simulink model "mars_rover_ex_3_22b"  (R2022b)
settings: Solver=ode23t  StartTime=0.0  StopTime=Rover.simStopTimeEx3  FixedStep=1e-2  MaxStep=0.05  RelTol=1e-3  AbsTol=1e-3  EnableMultiTasking=on
StartFcn:
  | setMechExplorerVisibility(bdroot,'hide');
  | mars_rover_ex3_sim_callback
StopFcn:
  | setMechExplorerVisibility(bdroot,'show');
model workspace (MATLAB code in the model file):
  | addpath("mars_rover_helpers");
  | % Load Rover Arm model for IK
  | mdlpath = ['mars_rover_data',filesep,'mars_rover_arm'];
  | load_system(mdlpath);
  | 
  | imdata = zeros(3,3,3);
  | 
  | % Temp
  | Kp_steer = 1;
  | Ki_steer = 1;
  | Kd_steer = 1;
  | 
  | Kp = 1;
  | Ki = 1;
  | Kd = 1;
values from neighbouring files (symbols this model uses):
  cam_base_angle = 0    [mars_rover_params.m]
  cam_target_angle = 20    [mars_rover_params.m]
  mapData = false(197,200)    [mars_rover_params.m]    (also in mars_rover_startup.m)
  roverPath = app.rover_path    [NavigateOnMars.m]    (also in mars_rover_params.m = rover_path1)
undefined symbols (not defined in the file or in its folder): Arm, armJointAng, armJointTrqs, cameraData, eeConfig, pose, Rover, sampleLocation, steerAng, steerTrqs, Terrain, vSpeed, Wheel1_G, Wheel2_G, Wheel3_G, Wheel4_G, Wheel5_G, Wheel6_G, wheelTrqs, wSpeeds, X, Y, Z
libraries: sm_lib x238, nesl_utility x80, slpidlib x3, simulink x3, simulink_extras x2, robotcorelib x1, robotalgslib x1
(part 1 of 9)
settings Model: PacingRate=4  Creator=The MathWorks, Inc.  LastModifiedBy=hupadhya
settings SolverCC: AutoScaleAbsTol=off  ZeroCrossAlgorithm=Adaptive  AlgebraicLoopSolver=TrustRegion  MinimalZcImpactIntegration=on  MaxZcPerStep=1
settings DataIOCC: MaxDataPoints=10000  SaveFormat=Array  ReturnWorkspaceOutputsName=sm_mars_rover_out_ex3
settings OptimizationCC: LifeSpan=inf
settings DebuggingCC: IgnoredZcDiagnostic=none  UnconnectedInputMsg=warning  UnconnectedOutputMsg=warning  UnconnectedLineMsg=warning  AllowSymbolicDim=off  SFUnexpectedBacktrackingDiag=warning  SFNoUnconditionalDefaultTransitionDiag=warning  SFExecutionAtInitializationDiag=none  SFMachineParentedDataDiag=warning  ArithmeticOperatorsInVariantConditions=warning
settings ModelReferenceCC: EnableRefExpFcnMdlSchedulingChecks=on
settings SFSimCC: SimUseLocalCustomCode=off  CustomCodeUndefinedFunction=UseInterfaceOnly
settings RTWCC: RTWUseLocalCustomCode=off  DLArmComputeVersion=19.05
settings CodeAppCC: StateflowObjectComments=on
settings GRTTargetCC: TargetLangStandard=C89/C90 (ANSI)
settings ConfigComp: CovMetricSettings=dw  CovSaveCumulativeToWorkspaceVar=on  CovSaveSingleToWorkspaceVar=on  CovExternalEMLEnable=off  CovSFcnEnable=off
settings SimscapeCC: SimscapeLogType=all  SimscapeLogSimulationStatistics=on  SimscapeLogName=simlog_sm_mars_rover  SimscapeLogLimitData=off  SimscapeLogDataHistory=10000
settings DiagnosticsConfigSet: SimMechanicsConflictingReferenceFrames=none
settings ExplorerConfigSet: InternalSimMechanicsExplorerSettings="<ExplorerConfiguration><canonicalview>default</canonicalview><AnimationSetting><BasePlaybackSpeed>1.0</BasePlaybackSpeed><PlaybackSpeedFactor>32.0</PlaybackSpeedFactor></AnimationSetting><TilePanel><TileInfo><Tiles Columns=\"1\" Count=\"1\" Rows=\"1\"><Column Weight=\"1\"/><Row Weight=\"1\"/><Tile Height=\"1\" Width=\"1\" X=\"0\" Y=\"0\"/></Tiles></TileInfo><SceneInfo><SceneViewer><BGColor><R>0.819607853889465332</R><G>0.709803938865661621</G><B>0.662745118141174316</B></BGColor><Camera><DoPerspective>off</DoPerspective><Position><X>20.000000787900472</X><Y>-8.56686066937523805</Y><Z>2.96310305518206007</Z></Position><Center><X>20.000000787900472</X><Y>19.6116538286981559</Y><Z>2.96310305518206007</Z></Center><Up><X>0</X><Y>-0</Y><Z>1</Z></Up><ViewLimDist>1</ViewLimDist><YLim>14.4034443168771542</YLim><XLim>20.6000000000000014</XLim></Camera></SceneViewer></SceneInfo></TilePanel><MechEditorPanel><Cameras><Camera><Id>Camera1</Id><Value><Name>Rover_Free_View</Name><NativeCamera><PositionKeyframeSet/><CenterKeyframeSet/><UpVectorKeyframeSet/></NativeCamera></Value></Camera><Camera><Id>Camera6</Id><Value><Name>Rover_Right_ViewA</Name><NativeCamera><PositionTrackingFeature>Mars_Rover.Rover_Plant_Model_And_Control.Rover.Chassis.Chasis_Camera_RightA.R</PositionTrackingFeature><CenterTrackingFeature>Mars_Rover.Rover_Plant_Model_And_Control.Rover.Chassis.Chasis_Camera_RightA.R</CenterTrackingFeature><UpVectorTrackingFeature>Mars_Rover.Rover_Plant_Model_And_Control.Rover.Chassis.Chasis_Camera_RightA.R</UpVectorTrackingFeature><CenterTrackingOrigin>off</CenterTrackingOrigin><CenterTrackingDirection>+X</CenterTrackingDirection><UpVectorTrackingDirection>+Z</UpVectorTrackingDirection></NativeCamera></Value></Camera><Camera><Id>Camera7</Id><Value><Name>Rover_Rear_View</Name><NativeCamera><PositionTrackingFeature>Mars_Rover.Rover_Plant_Model_And_Control.Rover.Chassis.Chasis_Camera_Rear.R</PositionTrackingFeature><CenterTrackingFeature>Mars_Rover.Rover_Plant_Model_And_Control.Rover.Chassis.Chasis_Camera_Rear.R</CenterTrackingFeature><UpVectorTrackingFeature>Mars_Rover.Rover_Plant_Model_And_Control.Rover.Chassis.Chasis_Camera_Rear.R</UpVectorTrackingFeature><CenterTrackingOrigin>off</CenterTrackingOrigin><CenterTrackingDirection>-Y</CenterTrackingDirection><UpVectorTrackingDirection>+Z</UpVectorTrackingDirection></NativeCamera></Value></Camera><Camera><Id>Camera8</Id><Value><Name>Rover_Top_View</Name><NativeCamera><PositionTrackingFeature>Mars_Rover.Rover_Plant_Model_And_Control.Rover.Chassis.Chasis_Camera_Top.R</PositionTrackingFeature><CenterTrackingFeature>Mars_Rover.Rover_Plant_Model_And_Control.Rover.Chassis.Chasis_Camera_Top.R</CenterTrackingFeature><UpVectorTrackingFeature>Mars_Rover.Rover_Plant_Model_And_Control.Rover.Chassis.Chasis_Camera_Top.R</UpVectorTrackingFeature><CenterTrackingOrigin>off</CenterTrackingOrigin><CenterTrackingDirection>-Z</CenterTrackingDirection><UpVectorTrackingDirection>+X</UpVectorTrackingDirection></NativeCamera></Value></Camera><Camera><Id>Camera9</Id><Value><Name>Rover_Right_ViewB</Name><NativeCamera><PositionTrackingFeature>Mars_Rover.Rover_Plant_Model_And_Control.Rover.Chassis.Chasis_Camera_RightB.R</PositionTrackingFeature><CenterTrackingFeature>Mars_Rover.Rover_Plant_Model_And_Control.Rover.Chassis.Chasis_Camera_RightB.R</CenterTrackingFeature><UpVectorTrackingFeature>Mars_Rover.Rover_Plant_Model_And_Control.Rover.Chassis.Chasis_Camera_RightB.R</UpVectorTrackingFeature><CenterTrackingOrigin>off</CenterTrackingOrigin><CenterTrackingDirection>+X</CenterTrackingDirection><UpVectorTrackingDirection>+Z</UpVectorTrackingDirection></NativeCamera></Value></Camera><Camera><Id>Camera10</Id><Value><Name>RoverNavCamL</Name><NativeCamera><PositionTrackingFeature>Mars_Rover.Rover_Plant_Model_And_Control.Rover.Camera.rsm_head_1_RIGID.CameraFrameL.F</PositionTrackingFeature><CenterTrackingFeature>Mars_Rover.Rover_Plant_Model_And_Control.Rover.Camera.rsm_head_1_RIGID.CameraFrameL.F</CenterTrackingFeature><UpVectorTrackingFeature>Mars_Rover.Rover_Plant_Model_And_Control.Rover.Camera.rsm_head_1_RIGID.CameraFrameL.F</UpVectorTrackingFeature><CenterTrackingOrigin>off</CenterTrackingOrigin><CenterTrackingDirection>+X</CenterTrackingDirection><UpVectorTrackingDirection>+Z</UpVectorTrackingDirection></NativeCamera></Value></Camera><Camera><Id>Camera11</Id><Value><Name>RoverNavCamR</Name><NativeCamera><PositionTrackingFeature>Mars_Rover.Rover_Plant_Model_And_Control.Rover.Camera.rsm_head_1_RIGID.CameraFrameR.F</PositionTrackingFeature><CenterTrackingFeature>Mars_Rover.Rover_Plant_Model_And_Control.Rover.Camera.rsm_head_1_RIGID.CameraFrameR.F</CenterTrackingFeature><UpVectorTrackingFeature>Mars_Rover.Rover_Plant_Model_And_Control.Rover.Camera.rsm_head_1_RIGID.CameraFrameR.F</UpVectorTrackingFeature><CenterTrackingOrigin>off</CenterTrackingOrigin><CenterTrackingDirection>+X</CenterTrackingDirection><UpVectorTrackingDirection>+Z</UpVectorTrackingDirection></NativeCamera></Value></Camera></Cameras><GfxPanelCameraMap/><VideoCreator><PlaybackSpeedRatio>8</PlaybackSpeedRatio><FrameRate>30</FrameRate><VideoFormat>MPEG-4</VideoFormat><FrameSize>[800 600]</FrameSize></VideoCreator></MechEditorPanel></ExplorerConfiguration>"

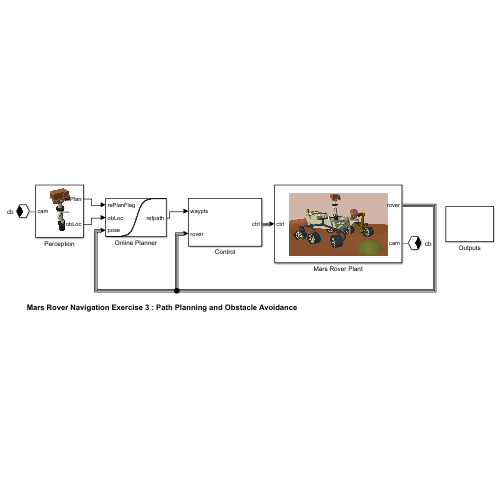
[thumbnail: Simulink's stored preview of the top-level diagram]
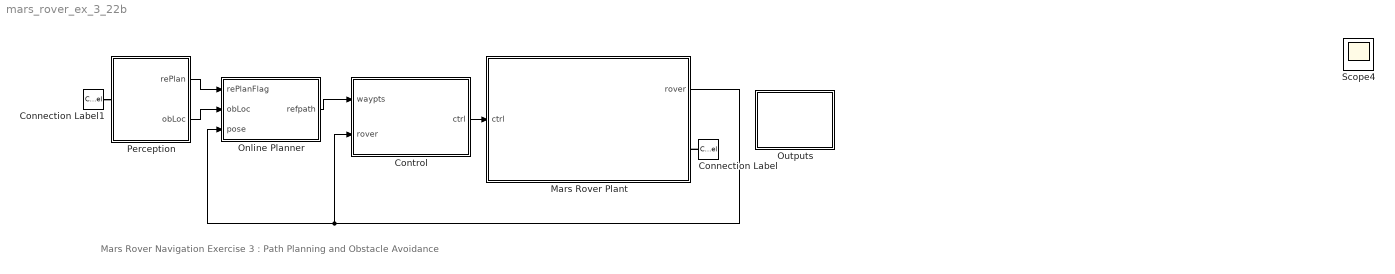
== system mars_rover_ex_3_22b ==
  note: Mars Rover Navigation Exercise 3 : Path Planning and Obstacle Avoidance
  Connection Label : ConnectionLabel  Label=cb
  Connection Label1 : ConnectionLabel  Label=cb
  Control : Subsystem
  Mars Rover Plant : Subsystem
      mask Display: image('$imagefile'); % Use "Edit Image" on toolstrip to change.
  Online Planner : Subsystem
      mask Display:
      | x = -5:0.01:5;
      | y = tanh(x);
      | plot(x,y)
  Outputs : Subsystem
  Perception : Subsystem
      mask Display: image('$imagefile'); % Use "Edit Image" on toolstrip to change.
  Scope4 : Scope
  wires:
  Mars Rover Plant/1(rover) -> Online Planner/3(pose), Control/2(rover)
  Control/1(ctrl) -> Mars Rover Plant/1(ctrl)
  Online Planner/1(refpath) -> Control/1(waypts)
  Perception/1(rePlan) -> Online Planner/1(rePlanFlag)
  Perception/2(obLoc) -> Online Planner/2(obLoc)
  connections:
  Connection Label/LConn1 -- Mars Rover Plant/RConn1
  Connection Label1/LConn1 -- Perception/LConn1

== system mars_rover_ex_3_22b/Control ==
  waypts : Inport
  rover : Inport  Port=2
  Bus Creator : BusCreator  Inputs=steerTrqs,wheelTrqs,armJointTrqs
  Bus Selector : BusSelector  OutputSignals=pose,vSpeed,steerAng,wSpeeds,sampleLocation,armJointAng
  Manipulator Control : Subsystem
  Rover Control : Subsystem
  ctrl : Outport
  wires:
  Bus Selector/3 -> Rover Control/4(ActSteerAng)  "<steerAng>"
  Bus Selector/6 -> Manipulator Control/2(ActJointAngles)  "<armJointAng>"
  Bus Selector/5 -> Manipulator Control/1(SampleLocation)  "<sampleLocation>"
  Bus Selector/2 -> Rover Control/3(vSpeed)  "<vSpeed>"
  Rover Control/2(WheelTrqs) -> Bus Creator/2  "wheelTrqs"
  Bus Selector/1 -> Rover Control/2(CurrentPose)  "<pose>"
  Bus Selector/4 -> Rover Control/5(ActWheelSpeed)  "<wSpeeds>"
  Rover Control/1(SteerTrqs) -> Bus Creator/1  "steerTrqs"
  Manipulator Control/1(y) -> Bus Creator/3  "armJointTrqs"
  rover/1 -> Bus Selector/1
  waypts/1 -> Rover Control/1(WayPts)
  Bus Creator/1 -> ctrl/1

== system mars_rover_ex_3_22b/Mars Rover Plant ==
  ctrl : Inport
  Bus Creator : BusCreator  Inputs=pose,vSpeed,steerAng,wSpeeds,armJointAng,sampleLocation
  Bus Selector : BusSelector  OutputSignals=steerTrqs,wheelTrqs,armJointTrqs
  DesRoverPathViz : Subsystem
  Manipulator Plant Model : Subsystem
      settings: PortSchema="{\"entries\":[{\"content\":{\"sides\":[{\"content\":{\"connectorIds\":[\"LConn1\",\"In1\"]},\"type\":\"ConnectorPlacement.EquallySpacedRectSide\",\"uuid\":\"1d5d5bba-8fe4-4512-81c9-941bf10e7a7e\"},{\"content\":{\"connectorIds\":[\"RConn1\",\"RConn2\",\"Out1\",\"Out2\"],\"side\":\"RIGHT\"},\"type\":\"ConnectorPlacement.EquallySpacedRectSide\",\"uuid\":\"9a182200-9de3-47d0-8b03-f46c5c0d90b9\"},{\"content\":{\"connectorIds\":[],\"side\":\"TOP\"},\"type\":\"ConnectorPlacement.EquallySpacedRectSide\",\"uuid\":\"d91c9a9a-8a5e-48c7-bbfb-96bbdec144af\"}]},\"type\":\"ConnectorPlacement.EquallySpacedConnector\",\"uuid\":\"893c2cf1-507c-408d-8167-3b555343645b\"}],\"packageUris\":[\"http://schema.mathworks.com/mf0/Connector/R2020b\"],\"version\":\"1.0\"}"
      mask Display:
      | image('RoverArmIcon.png'); % Use "Edit Image" on toolstrip to change.
      | 
      | color('black');
      | port_label('RConn',1,' sd','interpreter','tex')
      | port_label('LConn',1,' sb','interpreter','tex')
      | port_label('RConn',2,' armB','interpreter','tex')
      | port_label('output', 1, 'angles');
      | port_label('output', 2, 'sample');
      | port_label('input', 1, 'trqs');
  Rover Plant Model : Subsystem
      mask Display:
      | image('RoverIcon.PNG');
      | %image('$imagefile'); % Use "Edit Image" on toolstrip to change.
      | 
      | color('black');
      | port_label('LConn',1,' ref','interpreter','tex')
      | port_label('RConn',1,' armB','interpreter','tex')
      | port_label('RConn',2,' SD','interpreter','tex')
      | port_label('RConn',3,' CB','interpreter','tex')
      | port_label('output', 1, 'pose');
      | port_label('output', 2, 'vSpeed');
      | port_label('output', 3, 'sAng');
      | port_label('output', 4, 'wSpeed');
      | port_label('input', 1, 'sTrqs');
      | port_label('input', 2, 'wTrqs');
  cam : PMIOPort  Side=Right
  rover : Outport
  wires:
  Bus Selector/1 -> Rover Plant Model/1(Input)  "<steerTrqs>"
  Bus Selector/2 -> Rover Plant Model/2(Input1)  "<wheelTrqs>"
  Rover Plant Model/1(Pose) -> Bus Creator/1  "pose"
  Rover Plant Model/2(actRoverSpeed) -> Bus Creator/2  "vSpeed"
  Rover Plant Model/4(actWheelSpeeds) -> Bus Creator/4  "wSpeeds"
  Manipulator Plant Model/1(armJointAng) -> Bus Creator/5  "armJointAng"
  Manipulator Plant Model/2(sampleLocation) -> Bus Creator/6  "sampleLocation"
  Bus Selector/3 -> Manipulator Plant Model/1(Input)  "<armJointTrqs>"
  Bus Creator/1 -> rover/1
  Rover Plant Model/3(actSteerAng) -> Bus Creator/3  "steerAng"
  ctrl/1 -> Bus Selector/1
  connections:
  Rover Plant Model/LConn1 -- Manipulator Plant Model/LConn1 -- DesRoverPathViz/LConn1
  Rover Plant Model/RConn1 -- Manipulator Plant Model/RConn2
  Rover Plant Model/RConn2 -- Manipulator Plant Model/RConn1
  cam/RConn1 -- Rover Plant Model/RConn3

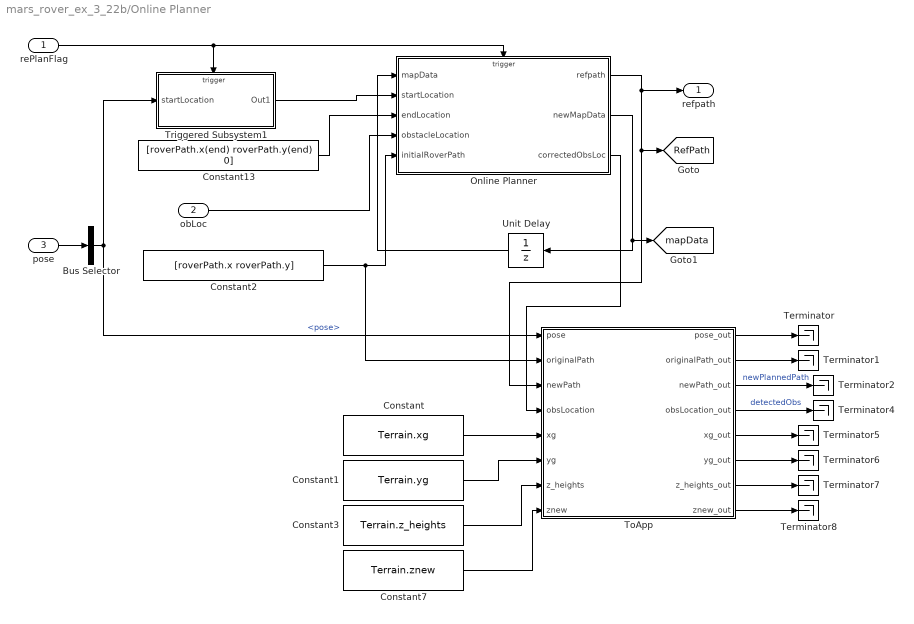
== system mars_rover_ex_3_22b/Online Planner ==
  rePlanFlag : Inport
  obLoc : Inport  Port=2
  pose : Inport  Port=3
  Bus Selector : BusSelector  OutputSignals=pose
  Constant : Constant  Value=Terrain.xg
  Constant1 : Constant  Value=Terrain.yg
  Constant13 : Constant  Value=[roverPath.x(end) roverPath.y(end) 0]
  Constant2 : Constant  Value=[roverPath.x roverPath.y]
  Constant3 : Constant  Value=Terrain.z_heights
  Constant7 : Constant  Value=Terrain.znew
  Online Planner : Subsystem
  Terminator{,1..2,4..8} (8 alike) : Terminator
  ToApp : MATLAB Function  TreatAsAtomicUnit=on
  Triggered Subsystem1 : Subsystem  TreatAsAtomicUnit=on
  Unit Delay : UnitDelay  InitialCondition=mapData  SampleTime=-1  HasFrameUpgradeWarning=on
  refpath : Outport
  tag scope: RefPath=global, mapData=global
  wires:
  Constant13/1 -> Online Planner/3(endLocation)
  Unit Delay/1 -> Online Planner/1(mapData)
  rePlanFlag/1 -> Triggered Subsystem1/Trigger, Online Planner/Trigger
  Triggered Subsystem1/1(Out1) -> Online Planner/2(startLocation)
  Online Planner/1(refpath) -> ToApp/3(newPath), [RefPath], refpath/1
  pose/1 -> Bus Selector/1
  Bus Selector/1 -> Triggered Subsystem1/1(startLocation), ToApp/1(pose)  "<pose>"
  Constant2/1 -> ToApp/2(originalPath), Online Planner/5(initialRoverPath)
  Online Planner/2(newMapData) -> Unit Delay/1, [mapData]
  ToApp/1(pose_out) -> Terminator/1
  ToApp/2(originalPath_out) -> Terminator1/1
  ToApp/3(newPath_out) -> Terminator2/1  "newPlannedPath"
  ToApp/4(obsLocation_out) -> Terminator4/1  "detectedObs"
  Constant/1 -> ToApp/5(xg)
  Constant1/1 -> ToApp/6(yg)
  Constant3/1 -> ToApp/7(z_heights)
  Constant7/1 -> ToApp/8(znew)
  ToApp/5(xg_out) -> Terminator5/1
  ToApp/6(yg_out) -> Terminator6/1
  ToApp/7(z_heights_out) -> Terminator7/1
  ToApp/8(znew_out) -> Terminator8/1
  obLoc/1 -> Online Planner/4(obstacleLocation)
  Online Planner/3(correctedObsLoc) -> ToApp/4(obsLocation)

== system mars_rover_ex_3_22b/Outputs ==
  Arm Outputs : Subsystem
  Rover Outputs : Subsystem

== system mars_rover_ex_3_22b/Perception ==
  AND : Logic  IconShape=distinctive  AllPortsSameDT=off  OutDataTypeStr=boolean
  Constant1 : Constant  Value=cam_base_angle
  Constant2 : Constant  Value=cam_target_angle
  MLFB : MATLAB Function  TreatAsAtomicUnit=on  mask{thresholdVal=0.58, roi=[0 0 0 0]}
      mask prompts: thresholdVal "Detection Threshold"; roi "Region of Interest"
  Memory : Memory  InitialCondition=[roverPath.x roverPath.y]
  Memory1 : Memory  InitialCondition=mapData
  NOT : Logic  Operator=NOT  IconShape=distinctive  AllPortsSameDT=off  OutDataTypeStr=boolean
  Pulse Generator : DiscretePulseGenerator  PulseType=Time based  Period=Rover.detection_sample_time
  Terminator1 : Terminator
  depthEstimation : MATLAB Function  TreatAsAtomicUnit=on
  navCamSubsystem : Subsystem
  rocksOnPath : MATLAB Function  TreatAsAtomicUnit=on
  sceneViewer : Subsystem
      settings: PortSchema="{\"entries\":[{\"content\":{\"sides\":[{\"content\":{\"connectorIds\":[\"LConn1\",\"LConn2\"]},\"type\":\"ConnectorPlacement.EquallySpacedRectSide\",\"uuid\":\"3e389f59-5740-42d0-b219-868887290247\"},{\"content\":{\"connectorIds\":[\"Out1\",\"Out2\"],\"side\":\"RIGHT\"},\"type\":\"ConnectorPlacement.EquallySpacedRectSide\",\"uuid\":\"8071baf0-f328-4328-afc3-7bbca75f94e9\"},{\"content\":{\"connectorIds\":[\"In1\"],\"side\":\"TOP\"},\"type\":\"ConnectorPlacement.EquallySpacedRectSide\",\"uuid\":\"389ad39b-6a15-4fbe-92ae-3d1bb225264a\"}]},\"type\":\"ConnectorPlacement.EquallySpacedConnector\",\"uuid\":\"9ad84bbc-3c32-4f8f-82ec-510eaa24821f\"}],\"packageUris\":[\"http://schema.mathworks.com/mf0/Connector/R2020b\"],\"version\":\"1.0\"}"
  cam : PMIOPort  Side=Left
  rePlan : Outport
  obLoc : Outport  Port=2
  wires:
  MLFB/1(bboxes) -> depthEstimation/3(in_bboxes)
  depthEstimation/2(obstacleWorldXYZ) -> rocksOnPath/1(obstacleWorldXYZ)
  depthEstimation/1(im_out) -> Terminator1/1
  [RoverTranslation] -> depthEstimation/4(rover_translation)
  [RoverOrientation] -> depthEstimation/5(rover_orientation)
  Constant1/1 -> depthEstimation/6(cam_base_angle)
  Constant2/1 -> depthEstimation/7(cam_target_angle)
  [RoverAtGoal] -> NOT/1
  NOT/1 -> AND/2
  rocksOnPath/1(rocksOnPath) -> obLoc/1
  rocksOnPath/2(rePlanFlag) -> rePlan/1
  Pulse Generator/1 -> AND/1
  [RefPath] -> Memory/1
  Memory/1 -> rocksOnPath/3(roverPath)
  [mapData] -> Memory1/1
  Memory1/1 -> rocksOnPath/4(mapData)
  depthEstimation/3(obstacleDistance) -> rocksOnPath/2(obstacleDistance)
  sceneViewer/1(im_left) -> depthEstimation/1(I_left), MLFB/1(image)
  AND/1 -> sceneViewer/1(captureFrame)
  sceneViewer/2(im_right) -> depthEstimation/2(I_right)
  connections:
  navCamSubsystem/RConn1 -- sceneViewer/LConn1
  sceneViewer/LConn2 -- navCamSubsystem/RConn2
  cam/RConn1 -- navCamSubsystem/LConn1

== system mars_rover_ex_3_22b/Control/Manipulator Control ==
  SampleLocation : Inport
  ActJointAngles : Inport  Port=2
  " Trajectory Planner" : Subsystem
  Add : Sum  Inputs=+-
  PID Control : slpidlib/PID Controller  Controller=PID  Form=Parallel  TimeDomain=Continuous-time  UseExternalTs=off  SampleTime=-1  IntegratorMethod=Forward Euler  FilterMethod=Forward Euler  ControllerParametersSource=internal  P=Arm.Kp_arm  I=Arm.Ki_arm  UseKiTs=off  D=Arm.Kd_arm  N=100  UseFilter=on  TunerSelectOption=Transfer Function Based (PID Tuner App)  InitialConditionSource=internal  InitialConditionForIntegrator=0  InitialConditionForFilter=0  DifferentiatorICPrevScaledInput=0  ExternalReset=none  TrackingMode=off  Kt=1  LimitOutput=off  SatLimitsSource=internal  UpperSaturationLimit=inf  LowerSaturationLimit=-inf  LinearizeAsGain=on  AntiWindupMode=none  Kb=1  LimitIntegrator=off  UpperIntegratorSaturationLimit=inf  LowerIntegratorSaturationLimit=-inf  POutMin=[]  POutMax=[]  IOutMin=[]  IOutMax=[]  DOutMin=[]  DOutMax=[]  NOutMin=[]  NOutMax=[]  SumOutMin=[]  SumOutMax=[]  SaturationOutMin=[]  SaturationOutMax=[]  PParamMin=[]  PParamMax=[]  IParamMin=[]  IParamMax=[]  DParamMin=[]  DParamMax=[]  NParamMin=[]  NParamMax=[]  KbParamMin=[]  KbParamMax=[]  KtParamMin=[]  KtParamMax=[]  KbOutMin=[]  KbOutMax=[]  KtOutMin=[]  KtOutMax=[]  IntegratorOutMin=[]  IntegratorOutMax=[]  FilterOutMin=[]  FilterOutMax=[]  SumI1OutMin=[]  SumI1OutMax=[]  SumI2OutMin=[]  SumI2OutMax=[]  SumI3OutMin=[]  SumI3OutMax=[]  SumI4OutMin=[]  SumI4OutMax=[]  SumDOutMin=[]  SumDOutMax=[]  DifferentiatorOutMin=[]  DifferentiatorOutMax=[]  FilterDiffOutCoefMin=[]  FilterDiffOutCoefMax=[]  ReciprocalOutMin=[]  ReciprocalOutMax=[]  SumDenOutMin=[]  SumDenOutMax=[]  SumNumOutMin=[]  SumNumOutMax=[]  DivideOutMin=[]  DivideOutMax=[]  UdiffTsProdOutMin=[]  UdiffTsProdOutMax=[]  NTsProdOutMin=[]  NTsProdOutMax=[]  UintegralTsProdOutMin=[]  UintegralTsProdOutMax=[]  UngainTsProdOutMin=[]  UngainTsProdOutMax=[]  ClampingZeroOutDataTypeStr=Inherit: Inherit via back propagation  ClampingZeroOutMin=[]  ClampingZeroOutMax=[]  FilterDenConstantOutDataTypeStr=Inherit: Inherit via back propagation  FilterDenConstantOutMin=[]  FilterDenConstantOutMax=[]  PCopyOutDataTypeStr=Inherit: Inherit via back propagation  PCopyOutMin=[]  PCopyOutMax=[]  NCopyOutDataTypeStr=Inherit: Inherit via back propagation  NCopyOutMin=[]  NCopyOutMax=[]  IntegratorContinuousStateAttributes=''  IntegratorStateMustResolveToSignalObject=off  IntegratorRTWStateStorageClass=Auto  FilterContinuousStateAttributes=''  FilterStateMustResolveToSignalObject=off  FilterRTWStateStorageClass=Auto  ParallelPVariant=InternalParameters  IdealPVariant=Disabled  IVariant=InternalParameters  DVariant=InternalParameters  IntegratorVariant=Continuous  SatVariant=Disabled  AWVariant=Passthrough  PCopyVariant=Disabled  TRVariant=Disabled  FdbkBlocksVariant=Forward  IdealPFdbkVariant=Disabled  SatFdbkVariant=Disabled  DerivativeFilterVariant=ContFilter  NVariant=InternalParameters  NCopyVariant=Disabled  FilterICVariant=InternalICsFilter  IntegratorICVariant=InternalICs  ExternalResetVariant=Disabled  TRSumVariant=Passthrough  SumFdbkVariant=Disabled  SumVariant=Sum_PID  TsampFilterVariant=InternalTs  TsampNgainVariant=Passthrough  TsampIntegralVariant=Passthrough  ExternalSaturationOutDataTypeStr=Inherit: Same as second input
  y : Outport
  tag scope: ActJointAngles=global, DesiredJointAngles=global, JointActuatorTrqs=global
  wires:
  PID Control/1 -> y/1, [JointActuatorTrqs]
  SampleLocation/1 -> " Trajectory Planner"/1(SampleLocation)
  ActJointAngles/1 -> Add/2, [ActJointAngles], " Trajectory Planner"/2(ActJointAngles)
  " Trajectory Planner"/1(DesiredJointAngles) -> Add/1, [DesiredJointAngles]
  Add/1 -> PID Control/1

== system mars_rover_ex_3_22b/Control/Rover Control ==
  WayPts : Inport
  CurrentPose : Inport  Port=2
  vSpeed : Inport  Port=3
  ActSteerAng : Inport  Port=4
  ActWheelSpeed : Inport  Port=5
  Rover Path Planning And Control : Subsystem
  Steering Controller : Subsystem
  Wheel Speed Controller : Subsystem
  SteerTrqs : Outport
  WheelTrqs : Outport  Port=2
  wires:
  Rover Path Planning And Control/2(DesWheelSpeeds) -> Wheel Speed Controller/1(DesWheelSpeeds)
  ActWheelSpeed/1 -> Wheel Speed Controller/2(ActWheelSpeed)
  Rover Path Planning And Control/1(DesSteerAngs) -> Steering Controller/1(DesSteerAng)
  CurrentPose/1 -> Rover Path Planning And Control/2(CurrentPose)
  Steering Controller/1(SteerTrqs) -> SteerTrqs/1
  ActSteerAng/1 -> Steering Controller/2(ActSteerAng)
  vSpeed/1 -> Rover Path Planning And Control/3(vSpeed)
  Wheel Speed Controller/1(WheelTrqs) -> WheelTrqs/1
  WayPts/1 -> Rover Path Planning And Control/1(WayPts)

== system mars_rover_ex_3_22b/Mars Rover Plant/DesRoverPathViz ==
  Cylindrical Solid : sm_lib/Body Elements/Cylindrical Solid  GraphicAmbientColor=[0.15 0.15 0.15 1.0]  BasedOnType=Density  CenterOfMass=[0 0 0]  CenterOfMassUnits=m  GraphicDiffuseColor=[0.4 0.4 1.0]  CylinderLength=0.1  CylinderLengthUnits=m  CylinderRadius=1  CylinderRadiusUnits=m  Density=1000  DensityUnits=kg/m^3  DoExposeReferenceFrame=on  GraphicEmissiveColor=[0.0 0.0 0.0 1.0]  ExportEntireGeometry=off  SerializedFrames=<Frames/>  MarkerShape=Sphere  MarkerSize=10  GraphicType=FromGeometry  InertiaType=CalculateFromGeometry  Mass=1  MassUnits=kg  MomentsOfInertia=[1 1 1]  MomentsOfInertiaUnits=kg*m^2  GraphicOpacity=0.5  ProductsOfInertia=[0 0 0]  ProductsOfInertiaUnits=kg*m^2  GraphicShininess=75  GraphicSpecularColor=[0.5 0.5 0.5 1.0]  GraphicVisPropType=SimpleVisualProperties
  Desired Path Viz : sm_lib/Curves and Surfaces/Point Cloud  CoordinatesMatrix=pointCloudPath  CoordinatesMatrixUnits=m  GraphicType=MarkerCloud  GraphicSphereRadius=0.05  GraphicSphereRadiusUnits=m  GraphicVisPropType=SimpleVisualProperties  GraphicDiffuseColor=[0 0 1]  GraphicOpacity=0.5  GraphicSpecularColor=[0.5 0.5 0.5 1.0]  GraphicAmbientColor=[0.15 0.15 0.15 1.0]  GraphicEmissiveColor=[0.0 0.0 0.0 1.0]  GraphicShininess=75
  Mechanism Configuration : sm_lib/Utilities/Mechanism Configuration  UniformGravity=Constant  GravityVector=[0 0 -3.7]  GravityUnits=m/s^2  LinearizationDelta=0.001  JointModeTransitionNonlinearIterations=2
  Rigid Transform1 : sm_lib/Frames and Transforms/Rigid Transform  TranslationMethod=Cartesian  TranslationStandardOffset=1.85  TranslationLengthUnit=m  TranslationStandardAxis=+Z  TranslationCartesianOffset=[roverPath.x(end) roverPath.y(end) roverPath.z(end)]  TranslationROffset=0  TranslationROffsetUnits=m  TranslationZOffset=0  TranslationZOffsetUnits=m  TranslationThetaOffset=0  TranslationThetaOffsetUnits=deg  RotationMethod=None  RotationAngleUnits=deg  RotationStandardAxis=+X  RotationAngle=90  RotationArbitraryAxis=[0 0 1]  FollAlignAxisA=+X  BaseAlignAxisA=+Y  FollAlignAxisB=+Y  BaseAlignAxisB=+Z  RotationSequenceAxes=FollowerAxes  RotationSequence=XYX  RotationSequenceAngles=[0 0 0]  RotationSequenceAnglesUnits=deg  RotationMatrix=[1 0 0; 0 1 0; 0 0 1]  Quaternion=[1 0 0 0]
  Rigid Transform6 : sm_lib/Frames and Transforms/Rigid Transform  TranslationMethod=Cartesian  TranslationStandardOffset=1.85  TranslationLengthUnit=m  TranslationStandardAxis=+Z  TranslationCartesianOffset=[0 0 roverPath.Offset_vis_z]  TranslationROffset=0  TranslationROffsetUnits=m  TranslationZOffset=0  TranslationZOffsetUnits=m  TranslationThetaOffset=0  TranslationThetaOffsetUnits=deg  RotationMethod=None  RotationAngleUnits=deg  RotationStandardAxis=+X  RotationAngle=90  RotationArbitraryAxis=[0 0 1]  FollAlignAxisA=+X  BaseAlignAxisA=+Y  FollAlignAxisB=+Y  BaseAlignAxisB=+Z  RotationSequenceAxes=FollowerAxes  RotationSequence=XYX  RotationSequenceAngles=[0 0 0]  RotationSequenceAnglesUnits=deg  RotationMatrix=[1 0 0; 0 1 0; 0 0 1]  Quaternion=[1 0 0 0]
  Solver Configuration : nesl_utility/Solver Configuration  PhysicalDomain=network_engine_domain  SubClassName=solver  LeftPortType=input  RightPortType=generic  Tones=[]  Harmonics=[]  SimulateNoise=off  Profile=off  UseLocalSampling=off  EnableSwitchedLinearOptims=on  FrequencyDomain=off  UseCCode=off  RelTol=0.001  AbsTol=1e-06  MinStep=1e-09  ToWorkspace=off  RevertToSquareIcSolve=off  NumHomotopyIterations=100  PhasorMode=off  PhasorModeNumHarmonics=1  ConsistencySolver=NEWTON_FTOL  IndexReductionMethod=DerivativeReplacement  DoDC=off  ResidualTolerance=1e-09  ConsistencyTolSource=GLOBAL  ConsistencyAbsTol=0.001  ConsistencyRelTol=0.001  ConsistencyTolFactor=0.001  UseLocalSolver=off  LocalSolverChoice=NE_BACKWARD_EULER_ADVANCER  ResolveIndetEquations=on  FunctionEvalNumThread=1  LocalSolverSampleTime=0.001  DoFixedCost=off  MaxNonlinIter=3  MaxModeIter=2  ComputeImpulses=off  ImpulseIterations=2  LinearAlgebra=auto  LinearAlgebraNumThread=0  EquationFormulation=NE_TIME_EF  DelaysMemoryBudget=1024  AutomaticFiltering=on  FilteringTimeConstant=0.001  PartitionStorageMethod=AS_NEEDED  PartitionMemoryBudget=1024  PartitionMethod=FAST
  World Frame : sm_lib/Frames and Transforms/World Frame
  R : PMIOPort  Side=Left
  connections:
  Rigid Transform1/LConn1 -- Rigid Transform6/RConn1 -- Desired Path Viz/LConn1
  Cylindrical Solid/RConn1 -- Rigid Transform1/RConn1
  R/RConn1 -- World Frame/RConn1 -- Solver Configuration/RConn1 -- Mechanism Configuration/RConn1 -- Rigid Transform6/LConn1

== system mars_rover_ex_3_22b/Mars Rover Plant/Manipulator Plant Model ==
  Input : Inport
  End Effector Sense : Subsystem
  Rover Arm : Subsystem
      mask Display: image('$imagefile'); % Use "Edit Image" on toolstrip to change.
  Sample Interaction Logic : Subsystem
      mask Display: image('$imagefile'); % Use "Edit Image" on toolstrip to change.
  Sample Loc Sense : Subsystem
  SampleGeneration : Subsystem
  RoverRef : PMIOPort  Side=Left
  SampleDrop : PMIOPort  Port=2  Side=Right
  ArmBase : PMIOPort  Port=3  Side=Right
  armJointAng : Outport
  sampleLocation : Outport  Port=2
  wires:
  Input/1 -> Rover Arm/1(ActuatorTrqs)
  Rover Arm/1(JointAngles) -> armJointAng/1
  Sample Loc Sense/1(SamplePos) -> sampleLocation/1
  connections:
  Sample Interaction Logic/RConn1 -- SampleDrop/RConn1
  End Effector Sense/RConn1 -- Sample Interaction Logic/LConn2 -- Rover Arm/RConn1
  Sample Interaction Logic/LConn3 -- Sample Loc Sense/RConn1
  ArmBase/RConn1 -- Sample Loc Sense/LConn1 -- End Effector Sense/LConn1 -- Rover Arm/LConn1
  SampleGeneration/LConn1 -- RoverRef/RConn1
  Sample Interaction Logic/LConn1 -- SampleGeneration/RConn1

== system mars_rover_ex_3_22b/Mars Rover Plant/Rover Plant Model ==
  Input : Inport
  Input1 : Inport  Port=2
  Rigid Terrain Surface : Subsystem
      mask Display: image('$imagefile'); % Use "Edit Image" on toolstrip to change.
  "Rover " : Subsystem
      settings: PortSchema="{\"entries\":[{\"content\":{\"sides\":[{\"content\":{\"connectorIds\":[\"In1\",\"In2\"]},\"type\":\"ConnectorPlacement.EquallySpacedRectSide\",\"uuid\":\"1e8a3e2b-b3ca-4467-863a-9c237d71771f\"},{\"content\":{\"connectorIds\":[\"RConn1\",\"Out1\",\"Out2\",\"RConn2\"],\"side\":\"RIGHT\"},\"type\":\"ConnectorPlacement.EquallySpacedRectSide\",\"uuid\":\"1c304fdb-ff64-4dc8-bd28-208b239a200a\"},{\"content\":{\"connectorIds\":[\"LConn1\",\"LConn2\",\"LConn3\"],\"side\":\"TOP\"},\"type\":\"ConnectorPlacement.EquallySpacedRectSide\",\"uuid\":\"6fd19973-5814-4525-bce6-20dd9c942e44\"},{\"content\":{\"connectorIds\":[],\"side\":\"BOTTOM\"},\"type\":\"ConnectorPlacement.EquallySpacedRectSide\",\"uuid\":\"ce53b395-dae7-4df5-bc94-fd3f2fb0670c\"}]},\"type\":\"ConnectorPlacement.EquallySpacedConnector\",\"uuid\":\"720db96a-3f3b-4ddd-a986-ea75ab459e47\"}],\"packageUris\":[\"http://schema.mathworks.com/mf0/Connector/R2020b\"],\"version\":\"1.0\"}"
      mask Display: image('$imagefile'); % Use "Edit Image" on toolstrip to change.
  Rover Pose Sensing : Subsystem
  Terminator : Terminator
  World Frame1 : sm_lib/Frames and Transforms/World Frame
  ArmB : PMIOPort  Side=Right
  SampleDropLoc : PMIOPort  Port=2  Side=Right
  B : PMIOPort  Port=3  Side=Left
  CB : PMIOPort  Port=4  Side=Right
  Pose : Outport
  actRoverSpeed : Outport  Port=2
  actSteerAng : Outport  Port=3
  actWheelSpeeds : Outport  Port=4
  wires:
  Rover Pose Sensing/3(vSpeed) -> actRoverSpeed/1
  "Rover "/1(ActSteerAng) -> actSteerAng/1
  "Rover "/2(ActWheelSpeeds) -> actWheelSpeeds/1
  Input/1 -> "Rover "/1(SteeringTrqs)
  Input1/1 -> "Rover "/2(WheelTrqs)
  Rover Pose Sensing/2(Pose) -> Pose/1
  Rover Pose Sensing/1(estimatedPose) -> Terminator/1
  connections:
  ArmB/RConn1 -- "Rover "/LConn1
  SampleDropLoc/RConn1 -- "Rover "/LConn2
  World Frame1/RConn1 -- Rigid Terrain Surface/RConn1
  Rigid Terrain Surface/LConn1 -- "Rover "/RConn2
  Rover Pose Sensing/LConn2 -- "Rover "/RConn1
  B/RConn1 -- Rover Pose Sensing/LConn1
  CB/RConn1 -- "Rover "/LConn3

== system mars_rover_ex_3_22b/Online Planner/Online Planner ==
  mapData : Inport  OutDataTypeStr=boolean
  startLocation : Inport  Port=2
  endLocation : Inport  Port=3
  obstacleLocation : Inport  Port=4
  initialRoverPath : Inport  Port=5
  Trigger : TriggerPort  VariantControl=(inherit)
  pathPlanner : MATLAB Function  TreatAsAtomicUnit=on
  refpath : Outport  InitialOutput=[roverPath.x roverPath.y]
  newMapData : Outport  Port=2  InitialOutput=mapData
  correctedObsLoc : Outport  Port=3  InitialOutput=zeros(100,3)
  wires:
  obstacleLocation/1 -> pathPlanner/4(obstacleLocation)
  mapData/1 -> pathPlanner/1(mapData)
  startLocation/1 -> pathPlanner/2(startLocation)
  pathPlanner/1(refpath) -> refpath/1
  endLocation/1 -> pathPlanner/3(endLocation)
  initialRoverPath/1 -> pathPlanner/5(initRoverPath)
  pathPlanner/2(newMapData) -> newMapData/1
  pathPlanner/3(correctedObsLoc) -> correctedObsLoc/1

== system mars_rover_ex_3_22b/Online Planner/Triggered Subsystem1 ==
  startLocation : Inport
  Trigger : TriggerPort  VariantControl=(inherit)
  Out1 : Outport
  wires:
  startLocation/1 -> Out1/1

== system mars_rover_ex_3_22b/Outputs/Arm Outputs ==
  ManipulatorJointActuatorTrqs : Scope  NumInputPorts=6
  ManipulatorJointAngles : Scope  NumInputPorts=6
  SelectSignal4 : Subsystem
  SelectSignal5 : Subsystem
  wires:
  SelectSignal4/5(Out4) -> ManipulatorJointAngles/5
  SelectSignal5/3(Out3) -> ManipulatorJointActuatorTrqs/3
  SelectSignal4/2(Out2) -> ManipulatorJointAngles/2
  SelectSignal4/1(Out1) -> ManipulatorJointAngles/1
  SelectSignal5/2(Out2) -> ManipulatorJointActuatorTrqs/2
  SelectSignal4/6(Out6) -> ManipulatorJointAngles/6
  SelectSignal5/4(Out5) -> ManipulatorJointActuatorTrqs/4
  SelectSignal4/3(Out3) -> ManipulatorJointAngles/3
  SelectSignal5/1(Out1) -> ManipulatorJointActuatorTrqs/1
  SelectSignal5/5(Out4) -> ManipulatorJointActuatorTrqs/5
  SelectSignal4/4(Out5) -> ManipulatorJointAngles/4
  [DesiredJointAngles] -> SelectSignal4/1(In1)
  [JointActuatorTrqs] -> SelectSignal5/1(In1)
  [ActJointAngles] -> SelectSignal4/2(In2)
  SelectSignal5/6(Out6) -> ManipulatorJointActuatorTrqs/6

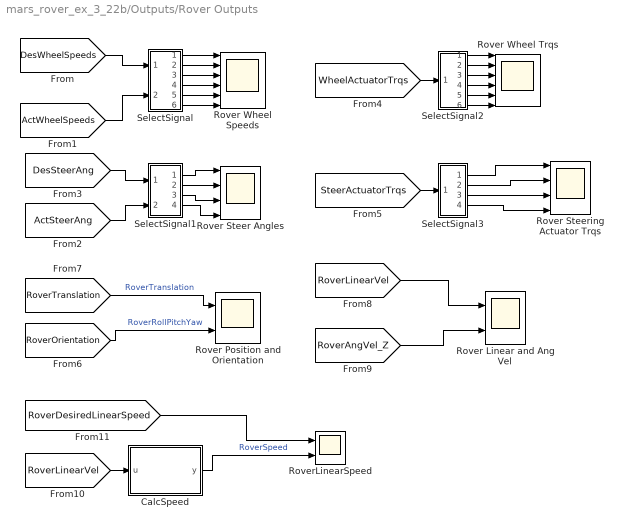
== system mars_rover_ex_3_22b/Outputs/Rover Outputs ==
  CalcSpeed : MATLAB Function  TreatAsAtomicUnit=on
  Rover Linear and Ang Vel : Scope  NumInputPorts=2
  Rover Position and Orientation : Scope  NumInputPorts=2
  Rover Steer Angles : Scope  NumInputPorts=4
  Rover Steering Actuator Trqs : Scope  NumInputPorts=4
  Rover Wheel Speeds : Scope  NumInputPorts=6
  Rover Wheel Trqs : Scope  NumInputPorts=6
  RoverLinearSpeed : Scope  NumInputPorts=2
  SelectSignal : Subsystem
  SelectSignal1 : Subsystem
  SelectSignal2 : Subsystem
  SelectSignal3 : Subsystem
  wires:
  CalcSpeed/1(y) -> RoverLinearSpeed/2  "RoverSpeed"
  SelectSignal3/1(Out1) -> Rover Steering Actuator Trqs/1
  [RoverLinearVel] -> CalcSpeed/1(u)
  [RoverAngVel_Z] -> Rover Linear and Ang Vel/2
  [RoverLinearVel] -> Rover Linear and Ang Vel/1
  [DesWheelSpeeds] -> SelectSignal/1(In1)
  SelectSignal2/4(Out4) -> Rover Wheel Trqs/4
  [WheelActuatorTrqs] -> SelectSignal2/1(In1)
  SelectSignal1/2(Out2) -> Rover Steer Angles/2
  [RoverTranslation] -> Rover Position and Orientation/1  "RoverTranslation"
  SelectSignal3/2(Out2) -> Rover Steering Actuator Trqs/2
  SelectSignal3/3(Out3) -> Rover Steering Actuator Trqs/3
  [DesSteerAng] -> SelectSignal1/1(In1)
  SelectSignal2/3(Out3) -> Rover Wheel Trqs/3
  [RoverOrientation] -> Rover Position and Orientation/2  "RoverRollPitchYaw"
  SelectSignal3/4(Out5) -> Rover Steering Actuator Trqs/4
  SelectSignal2/6(Out6) -> Rover Wheel Trqs/6
  SelectSignal/3(Out3) -> Rover Wheel Speeds/3
  SelectSignal2/5(Out5) -> Rover Wheel Trqs/5
  SelectSignal/1(Out1) -> Rover Wheel Speeds/1
  SelectSignal/6(Out6) -> Rover Wheel Speeds/6
  [ActWheelSpeeds] -> SelectSignal/2(In2)
  SelectSignal2/1(Out1) -> Rover Wheel Trqs/1
  SelectSignal1/4(Out5) -> Rover Steer Angles/4
  [ActSteerAng] -> SelectSignal1/2(In2)
  SelectSignal/2(Out2) -> Rover Wheel Speeds/2
  [SteerActuatorTrqs] -> SelectSignal3/1(In1)
  SelectSignal/5(Out4) -> Rover Wheel Speeds/5
  SelectSignal2/2(Out2) -> Rover Wheel Trqs/2
  SelectSignal/4(Out5) -> Rover Wheel Speeds/4
  SelectSignal1/1(Out1) -> Rover Steer Angles/1
  SelectSignal1/3(Out3) -> Rover Steer Angles/3
  [RoverDesiredLinearSpeed] -> RoverLinearSpeed/1

== system mars_rover_ex_3_22b/Perception/navCamSubsystem ==
  Constant : Constant  Value=cam_base_angle
  Revolute Joint5 : sm_lib/Joints/Revolute Joint  JointMode=Normal  SenseConstraintForce=off  SenseConstraintForceX=off  SenseConstraintForceY=off  SenseConstraintForceZ=off  SenseConstraintTorque=off  SenseConstraintTorqueX=off  SenseConstraintTorqueY=off  SenseConstraintTorqueZ=off  SenseTotalForce=off  SenseTotalForceX=off  SenseTotalForceY=off  SenseTotalForceZ=off  SenseTotalTorque=off  SenseTotalTorqueX=off  SenseTotalTorqueY=off  SenseTotalTorqueZ=off  CompositeWrenchDir=FollowerOnBase  CompositeWrenchFrame=BaseFrame  EquilibriumPosition=0  EquilibriumPositionUnits=deg  SpringStiffness=0  SpringStiffnessUnits=N*m/deg  DampingCoefficient=0  DampingCoefficientUnits=N*m/(deg/s)  TorqueActuationMode=ComputedTorque  MotionActuationMode=InputMotion  SensePosition=off  SenseVelocity=off  SenseAcceleration=off  SenseTorqueForce=off  SenseLowerLimitTorqueForce=off  SenseUpperLimitTorqueForce=off  LowerLimitSpecify=off  LowerLimitBound=-90  LowerLimitBoundUnits=deg  LowerLimitStiffness=1e4  LowerLimitStiffnessUnits=N*m/deg  LowerLimitDamping=10  LowerLimitDampingUnits=N*m/(deg/s)  LowerLimitTransitionRegionWidth=0.1  LowerLimitTransitionRegionWidthUnits=deg  UpperLimitSpecify=off  UpperLimitBound=90  UpperLimitBoundUnits=deg  UpperLimitStiffness=1e4  UpperLimitStiffnessUnits=N*m/deg  UpperLimitDamping=10  UpperLimitDampingUnits=N*m/(deg/s)  UpperLimitTransitionRegionWidth=0.1  UpperLimitTransitionRegionWidthUnits=deg  PositionTargetSpecify=off  PositionTargetPriority=High  PositionTargetValue=0  PositionTargetValueUnits=deg  VelocityTargetSpecify=off  VelocityTargetPriority=High  VelocityTargetValue=0  VelocityTargetValueUnits=deg/s
  Rigid Transform1 : sm_lib/Frames and Transforms/Rigid Transform  TranslationMethod=None  TranslationStandardOffset=0  TranslationLengthUnit=m  TranslationStandardAxis=+Z  TranslationCartesianOffset=[0 0 0]  TranslationROffset=0  TranslationROffsetUnits=m  TranslationZOffset=0  TranslationZOffsetUnits=m  TranslationThetaOffset=0  TranslationThetaOffsetUnits=deg  RotationMethod=StandardAxis  RotationAngleUnits=deg  RotationStandardAxis=+X  RotationAngle=90  RotationArbitraryAxis=[0 0 1]  FollAlignAxisA=+X  BaseAlignAxisA=+Y  FollAlignAxisB=+Y  BaseAlignAxisB=+Z  RotationSequenceAxes=FollowerAxes  RotationSequence=XYX  RotationSequenceAngles=[0 0 0]  RotationSequenceAnglesUnits=deg  RotationMatrix=[1 0 0; 0 1 0; 0 0 1]  Quaternion=[1 0 0 0]
  Rigid Transform2 : sm_lib/Frames and Transforms/Rigid Transform  TranslationMethod=None  TranslationStandardOffset=0  TranslationLengthUnit=m  TranslationStandardAxis=+Z  TranslationCartesianOffset=[0 0 0]  TranslationROffset=0  TranslationROffsetUnits=m  TranslationZOffset=0  TranslationZOffsetUnits=m  TranslationThetaOffset=0  TranslationThetaOffsetUnits=deg  RotationMethod=StandardAxis  RotationAngleUnits=deg  RotationStandardAxis=+X  RotationAngle=-90  RotationArbitraryAxis=[0 0 1]  FollAlignAxisA=+X  BaseAlignAxisA=+Y  FollAlignAxisB=+Y  BaseAlignAxisB=+Z  RotationSequenceAxes=FollowerAxes  RotationSequence=XYX  RotationSequenceAngles=[0 0 0]  RotationSequenceAnglesUnits=deg  RotationMatrix=[1 0 0; 0 1 0; 0 0 1]  Quaternion=[1 0 0 0]
  Simulink-PS Converter : nesl_utility/Simulink-PS Converter  PhysicalDomain=network_engine_domain  SubClassName=ps_input  LeftPortType=input  RightPortType=output  PseudoPeriodic=off  Frequencies=[]  NoiseDistribution=none  NoiseParameters=[]  Unit=deg  AffineConversion=off  FilteringAndDerivatives=filter  SimscapeFilterOrder=2  InputFilterTimeConstant=0.001  UdotUserProvided=0
  rsm_base_1_RIGID : Subsystem
  rsm_head_1_RIGID : Subsystem
  rsm_lower_mast_2_RIGID : Subsystem
  rsm_outer_ring_1_RIGID : Subsystem
  rsm_upper_mast_1_RIGID : Subsystem
  RightNavCam : PMIOPort  Side=Right
  LeftNavCam : PMIOPort  Port=2  Side=Right
  CB : PMIOPort  Port=3  Side=Left
  wires:
  Constant/1 -> Simulink-PS Converter/1
  connections:
  CB/RConn1 -- Rigid Transform1/LConn1
  Revolute Joint5/RConn1 -- Rigid Transform2/LConn1
  rsm_lower_mast_2_RIGID/RConn1 -- rsm_outer_ring_1_RIGID/LConn2
  Rigid Transform2/RConn1 -- rsm_base_1_RIGID/LConn1
  LeftNavCam/RConn1 -- rsm_head_1_RIGID/RConn2
  rsm_outer_ring_1_RIGID/LConn1 -- rsm_upper_mast_1_RIGID/LConn1
  rsm_lower_mast_2_RIGID/LConn1 -- rsm_base_1_RIGID/LConn2
  Revolute Joint5/LConn2 -- Simulink-PS Converter/RConn1
  Rigid Transform1/RConn1 -- Revolute Joint5/LConn1
  rsm_head_1_RIGID/LConn1 -- rsm_upper_mast_1_RIGID/RConn1
  rsm_head_1_RIGID/RConn1 -- RightNavCam/RConn1

== system mars_rover_ex_3_22b/Perception/sceneViewer ==
  captureFrame : Inport
  Left : Subsystem
  Right : Subsystem
  Stereo_Left : Subsystem
  Stereo_Right : Subsystem
  rightCamFrame : PMIOPort  Side=Left
  leftCamFrame : PMIOPort  Port=2  Side=Left
  im_left : Outport
  im_right : Outport  Port=2
  wires:
  Stereo_Right/1(im_right) -> im_right/1
  captureFrame/1 -> Stereo_Right/1(Input), Stereo_Left/1(Input)
  Stereo_Left/1(im_left) -> im_left/1
  connections:
  Stereo_Right/LConn1 -- rightCamFrame/RConn1 -- Right/RConn1
  Stereo_Left/LConn1 -- Left/RConn1 -- leftCamFrame/RConn1

== system mars_rover_ex_3_22b/Control/Manipulator Control/ Trajectory Planner ==
  SampleLocation : Inport
  ActJointAngles : Inport  Port=2
  Constant : Constant  Value="[-2.2294 -125.2918   50.0575 -175.3493  177.7706  180.0000]"
  Delay : Delay
  Delay1 : Delay  DelayLength=35
  Planner Subsystem : Subsystem
  SampleDropOffCmdLogic : Subsystem
  SampleLoc wrt arm base : Subsystem
  SamplePickUpCmdLogic : Subsystem
  Stop Simulation : Stop
  Switch : Switch  Criteria=u2 > Threshold  SaturateOnIntegerOverflow=off  InputSameDT=off
  DesiredJointAngles : Outport
  tag scope: SampleDropOffFlag=global, SamplePickFlag=global
  wires:
  Switch/1 -> DesiredJointAngles/1
  Constant/1 -> Switch/3
  SampleDropOffCmdLogic/1(Out1) -> [SampleDropOffFlag]
  SamplePickUpCmdLogic/1(Out1) -> [SamplePickFlag]
  Delay/1 -> Switch/2
  ActJointAngles/1 -> Planner Subsystem/1(ActJointAngles)
  SampleLoc wrt arm base/1(SamplePos) -> Planner Subsystem/2(SamplePosition)
  Planner Subsystem/2(SamplePickCmd) -> SamplePickUpCmdLogic/1(u)
  Planner Subsystem/3(SampleDropCmd) -> SampleDropOffCmdLogic/1(u)
  [samplePickedSense] -> Planner Subsystem/3(IsSamplePicked)
  [sampleStoredSense] -> Planner Subsystem/4(IsSampleCollected)
  Planner Subsystem/1(DesJointAngles) -> Switch/1
  Planner Subsystem/4(stop) -> Stop Simulation/1
  [RoverAtGoal] -> Delay1/1
  Delay1/1 -> Planner Subsystem/Enable, Delay/1, SampleLoc wrt arm base/1(Enable)
  SampleLocation/1 -> SampleLoc wrt arm base/2(SampleLoc)

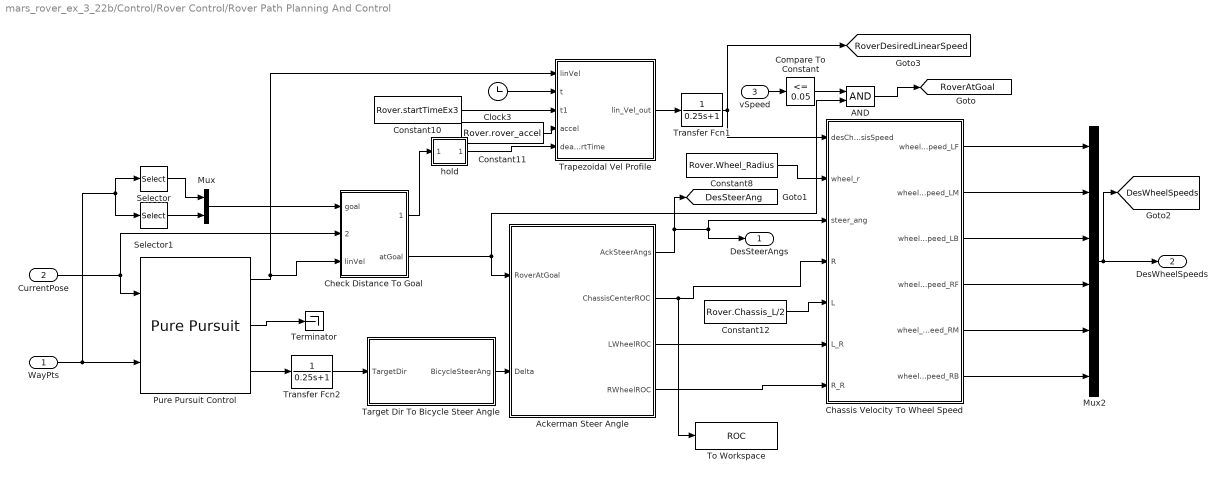
== system mars_rover_ex_3_22b/Control/Rover Control/Rover Path Planning And Control ==
  WayPts : Inport
  CurrentPose : Inport  Port=2
  vSpeed : Inport  Port=3
  AND : Logic  IconShape=distinctive  AllPortsSameDT=off  OutDataTypeStr=boolean
  Ackerman Steer Angle : Subsystem
  Chassis Velocity To Wheel Speed : MATLAB Function  TreatAsAtomicUnit=on
  Check Distance To Goal : Subsystem
  Clock3 : Clock
  Compare To Constant : simulink/Logic and Bit Operations/Compare To Constant  relop=<=  const=0.05  OutDataTypeStr=boolean
  Constant10 : Constant  Value=Rover.startTimeEx3
  Constant11 : Constant  Value=Rover.rover_accel
  Constant12 : Constant  Value=Rover.Chassis_L/2
  Constant8 : Constant  Value=Rover.Wheel_Radius
  Mux : Mux  Inputs=2
  Mux2 : Mux  Inputs=6
  Pure Pursuit Control : robotalgslib/Pure Pursuit  DesiredLinearVelocity=0.03  MaxAngularVelocity=0.01  LookaheadDistance=0.75  TargetDirPort=on  SimulateUsing=Code generation
  Selector : Selector  NumberOfDimensions=2  InputPortWidth=6  IndexOptions=Index vector (dialog),Index vector (dialog)  Indices=length(roverPath.x),1  OutputSizes=1,1
  Selector1 : Selector  NumberOfDimensions=2  InputPortWidth=6  IndexOptions=Index vector (dialog),Index vector (dialog)  Indices=length(roverPath.x),2  OutputSizes=1,1
  Target Dir To Bicycle Steer Angle : Subsystem  mask{L=Rover.Chassis_L/2, ld=0.75}
      mask prompts: L "Bicycle length"; ld "Lookahead distance"
      mask TypeOptions L: Bicycle length/Value
      mask TypeOptions ld: Lookahead distance/Value
  Terminator : Terminator
  To Workspace : ToWorkspace  VariableName=ROC  SampleTime=-1
  Transfer Fcn1 : TransferFcn  Denominator=[0.25 1]
  Transfer Fcn2 : TransferFcn  Denominator=[0.25 1]
  Trapezoidal Vel Profile : MATLAB Function  TreatAsAtomicUnit=on
  hold : Subsystem
  DesSteerAngs : Outport
  DesWheelSpeeds : Outport  Port=2
  tag scope: DesSteerAng=global, DesWheelSpeeds=global, RoverAtGoal=global, RoverDesiredLinearSpeed=global
  wires:
  Mux/1 -> Check Distance To Goal/1(goal)
  CurrentPose/1 -> Pure Pursuit Control/1, Check Distance To Goal/2(currentPose)
  Check Distance To Goal/2(atGoal) -> Ackerman Steer Angle/1(RoverAtGoal), AND/2
  Clock3/1 -> Trapezoidal Vel Profile/2(t)
  Constant10/1 -> Trapezoidal Vel Profile/3(t1)
  Constant11/1 -> Trapezoidal Vel Profile/4(accel)
  Constant8/1 -> Chassis Velocity To Wheel Speed/2(wheel_r)
  Constant12/1 -> Chassis Velocity To Wheel Speed/5(L)
  Mux2/1 -> [DesWheelSpeeds], DesWheelSpeeds/1
  Check Distance To Goal/1(deAccel) -> hold/1(In1)
  hold/1(Out1) -> Trapezoidal Vel Profile/5(deaccelStartTime)
  Ackerman Steer Angle/1(AckSteerAngs) -> [DesSteerAng], Chassis Velocity To Wheel Speed/3(steer_ang), DesSteerAngs/1
  Target Dir To Bicycle Steer Angle/1(BicycleSteerAng) -> Ackerman Steer Angle/2(Delta)
  Ackerman Steer Angle/2(ChassisCenterROC) -> To Workspace/1, Chassis Velocity To Wheel Speed/4(R)
  Ackerman Steer Angle/3(LWheelROC) -> Chassis Velocity To Wheel Speed/6(L_R)
  Ackerman Steer Angle/4(RWheelROC) -> Chassis Velocity To Wheel Speed/7(R_R)
  Pure Pursuit Control/2 -> Terminator/1
  Compare To Constant/1 -> AND/1
  AND/1 -> [RoverAtGoal]
  Chassis Velocity To Wheel Speed/1(wheel_speed_LF) -> Mux2/1
  Chassis Velocity To Wheel Speed/2(wheel_speed_LM) -> Mux2/2
  Chassis Velocity To Wheel Speed/3(wheel_speed_LB) -> Mux2/3
  Chassis Velocity To Wheel Speed/4(wheel_speed_RF) -> Mux2/4
  Chassis Velocity To Wheel Speed/5(wheel_speed_RM) -> Mux2/5
  Chassis Velocity To Wheel Speed/6(wheel_speed_RB) -> Mux2/6
  Trapezoidal Vel Profile/1(lin_Vel_out) -> Transfer Fcn1/1
  vSpeed/1 -> Compare To Constant/1
  Transfer Fcn1/1 -> [RoverDesiredLinearSpeed], Chassis Velocity To Wheel Speed/1(desChassisSpeed)
  WayPts/1 -> Pure Pursuit Control/2, Selector/1, Selector1/1
  Pure Pursuit Control/3 -> Transfer Fcn2/1
  Pure Pursuit Control/1 -> Trapezoidal Vel Profile/1(linVel), Check Distance To Goal/3(linVel)
  Transfer Fcn2/1 -> Target Dir To Bicycle Steer Angle/1(TargetDir)
  Selector/1 -> Mux/1
  Selector1/1 -> Mux/2
